simulink model "Furuta_Template_s"  (Simulink 10.0)
settings: Solver=ode4  StartTime=0.0  StopTime=50  FixedStep=0.0001  RelTol=1e-8  EnableMultiTasking=on
values from neighbouring files (symbols this model uses):
  b1 = 10^-4    (= 0.0001)    [SystemParameters.m]    (also in changeable_parameters.m)
  b2 = 2.8*(10^-4)    (= 0.00028)    [SystemParameters.m]    (also in changeable_parameters.m)
  g = 9.8    [SystemParameters.m]
  J2Hat = J2 + M2*((l2)^2)    (= 0.0055028)    [SystemParameters.m]
  JNotHat = J1Hat + M2*((L1)^2)    (= 0.0373463)    [SystemParameters.m]
  Km = 0.09    [SystemParameters.m]    (also in changeable_parameters.m)
  L = 0.005    [SystemParameters.m]    (also in changeable_parameters.m)
  L1 = 0.278    [SystemParameters.m]    (also in changeable_parameters.m)
  l2 = 0.148    [SystemParameters.m]    (also in changeable_parameters.m)
  M2 = 0.075    [SystemParameters.m]
  R = 7.8    [SystemParameters.m]    (also in changeable_parameters.m = B_mod'*Rh*Rh*B_mod)
  theta2_Init = pi +0.1    (= 3.24159265359)    [SystemParameters.m]
settings Model: Creator=mecmg  LastModifiedBy=Owner
settings DataIOCC: LimitDataPoints=on  SignalLoggingSaveFormat=ModelDataLogs
settings OptimizationCC: ExpressionDepthLimit=2147483647
settings DebuggingCC: SolverPrmCheckMsg=warning  FcnCallInpInsideContextMsg=warning  StateNameClashWarn=warning
settings GRTTargetCC: GeneratePreprocessorConditionals=Disable all
settings ConfigComp: CovExternalEMLEnable=off

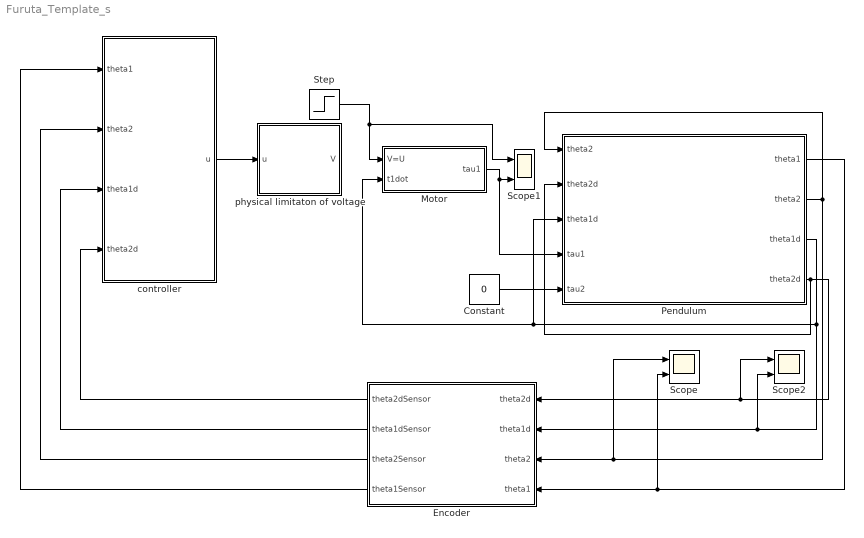
== system Furuta_Template_s ==
  Constant : Constant  Value=0  VectorParams1D=off
  Encoder : Subsystem
  Motor : Subsystem
  Pendulum : Subsystem
  Scope : Scope  NumInputPorts=2
  Scope1 : Scope  NumInputPorts=2
  Scope2 : Scope  NumInputPorts=2
  Step : Step  After=-10  SampleTime=0
  controller : Subsystem
  physical limitaton of voltage : Subsystem
  wires:
  controller/1(u) -> physical limitaton of voltage/1(u)
  Encoder/1(theta2dSensor) -> controller/4(theta2d)
  Encoder/4(theta1Sensor) -> controller/1(theta1)
  Encoder/2(theta1dSensor) -> controller/3(theta1d)
  Encoder/3(theta2Sensor) -> controller/2(theta2)
  Pendulum/2(theta2) -> Encoder/3(theta2), Scope/1, Pendulum/1("theta2  ")
  Pendulum/1(theta1) -> Encoder/4(theta1), Scope/2
  Pendulum/3(theta1d) -> Motor/2(t1dot), Pendulum/3("theta1d "), Scope2/2, Encoder/2(theta1d)
  Pendulum/4(theta2d) -> Pendulum/2("theta2d "), Scope2/1, Encoder/1(theta2d)
  Constant/1 -> Pendulum/5(tau2)
  Step/1 -> Scope1/1, Motor/1(V=U)
  Motor/1(tau1) -> Scope1/2, Pendulum/4(tau1)

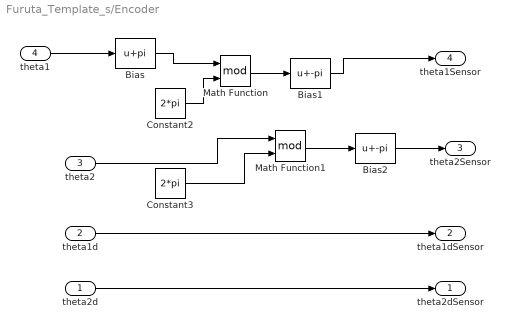
== system Furuta_Template_s/Encoder ==
  theta2d : Inport
  theta1d : Inport  Port=2
  theta2 : Inport  Port=3
  theta1 : Inport  Port=4
  Bias : Bias  Bias=pi
  Bias1 : Bias  Bias=-pi
  Bias2 : Bias  Bias=-pi
  Constant2 : Constant  Value=2*pi
  Constant3 : Constant  Value=2*pi
  Math Function : Math  Operator=mod  SignedPower=off  SaturateOnIntegerOverflow=on
  Math Function1 : Math  Operator=mod  SignedPower=off  SaturateOnIntegerOverflow=on
  theta2dSensor : Outport
  theta1dSensor : Outport  Port=2
  theta2Sensor : Outport  Port=3
  theta1Sensor : Outport  Port=4
  wires:
  theta1d/1 -> theta1dSensor/1
  theta2d/1 -> theta2dSensor/1
  theta1/1 -> Bias/1
  Constant2/1 -> Math Function/2
  Math Function/1 -> Bias1/1
  Math Function1/1 -> Bias2/1
  Constant3/1 -> Math Function1/2
  theta2/1 -> Math Function1/1
  Bias/1 -> Math Function/1
  Bias1/1 -> theta1Sensor/1
  Bias2/1 -> theta2Sensor/1

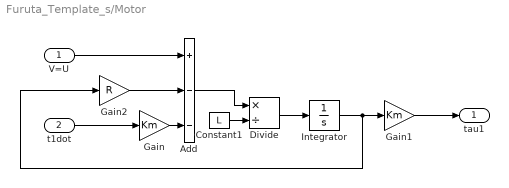
== system Furuta_Template_s/Motor ==
  V=U : Inport
  t1dot : Inport  Port=2
  Add : Sum  Inputs=+--
  Constant1 : Constant  Value=L
  Divide : Product  Inputs=*/
  Gain : Gain  Gain=Km
  Gain1 : Gain  Gain=Km
  Gain2 : Gain  Gain=R
  Integrator : Integrator
  tau1 : Outport
  wires:
  V=U/1 -> Add/1
  Gain2/1 -> Add/2
  t1dot/1 -> Gain/1
  Gain/1 -> Add/3
  Add/1 -> Divide/1
  Constant1/1 -> Divide/2
  Divide/1 -> Integrator/1
  Integrator/1 -> Gain2/1, Gain1/1
  Gain1/1 -> tau1/1

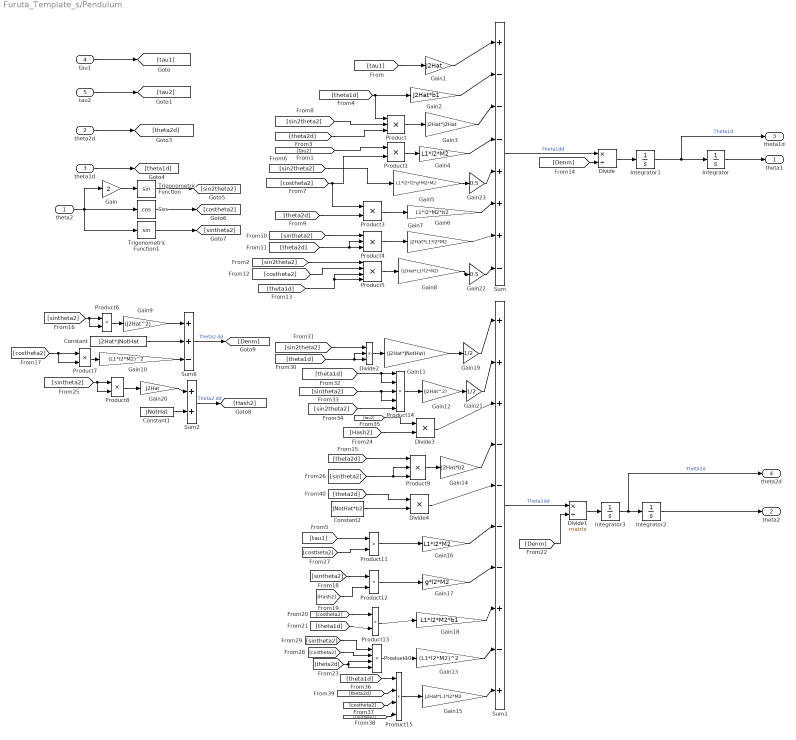
== system Furuta_Template_s/Pendulum ==
  "theta2  " : Inport
  "theta2d " : Inport  Port=2
  "theta1d " : Inport  Port=3
  tau1 : Inport  Port=4
  tau2 : Inport  Port=5
  Constant : Constant  Value=J2Hat*JNotHat
  Constant1 : Constant  Value=JNotHat
  Constant2 : Constant  Value=JNotHat*b2
  Cos : Trigonometry  Operator=cos
  Divide : Product  Inputs=*/
  Divide1 : Product  Inputs=*/  Multiplication=Matrix(*)
  Divide2 : Product  Inputs=***
  Divide3 : Product
  Divide4 : Product
  Gain : Gain  Gain=2
  Gain1 : Gain  Gain=J2Hat
  Gain10 : Gain  Gain=(L1*l2*M2)^2
  Gain11 : Gain  Gain=(J2Hat*JNotHat)
  Gain12 : Gain  Gain=(J2Hat^2)
  Gain13 : Gain  Gain=(L1*l2*M2)^2
  Gain14 : Gain  Gain=J2Hat*b2
  Gain15 : Gain  Gain=J2Hat*L1*l2*M2
  Gain16 : Gain  Gain=L1*l2*M2
  Gain17 : Gain  Gain=g*l2*M2
  Gain18 : Gain  Gain=L1*l2*M2*b1
  Gain19 : Gain  Gain=1/2
  Gain2 : Gain  Gain=J2Hat*b1
  Gain20 : Gain  Gain=J2Hat
  Gain21 : Gain  Gain=1/2
  Gain22 : Gain  Gain=0.5
  Gain23 : Gain  Gain=0.5
  Gain3 : Gain  Gain=J2Hat*J2Hat
  Gain4 : Gain  Gain=L1*l2*M2
  Gain5 : Gain  Gain=L1*l2*l2*g*M2*M2
  Gain6 : Gain  Gain=L1*l2*M2*b2
  Gain7 : Gain  Gain=J2Hat*L1*l2*M2
  Gain8 : Gain  Gain=(J2Hat*L1*l2*M2)
  Gain9 : Gain  Gain=(J2Hat^2)
  Integrator : Integrator  UpperSaturationLimit=pi  LowerSaturationLimit=-pi
  Integrator1 : Integrator
  Integrator2 : Integrator  InitialCondition=theta2_Init  UpperSaturationLimit=pi  LowerSaturationLimit=-pi
  Integrator3 : Integrator
  Product : Product  Inputs=3
  Product{1,3,6..8,11..13} (8 alike) : Product
  Product10 : Product  Inputs=4
  Product14 : Product  Inputs=5
  Product15 : Product  Inputs=4
  Product4 : Product  Inputs=3
  Product5 : Product  Inputs=4
  Product9 : Product  Inputs=3
  Sum : Sum  Inputs=|+---+++-
  Sum1 : Sum  Inputs=|+++----+-+
  Sum2 : Sum
  Sum6 : Sum  Inputs=++-
  Trigonometric Function : Trigonometry
  Trigonometric Function1 : Trigonometry
  theta1 : Outport
  theta2 : Outport  Port=2
  theta1d : Outport  Port=3
  theta2d : Outport  Port=4
  wires:
  Integrator1/1 -> Integrator/1, theta1d/1  "Theta1d"
  Integrator/1 -> theta1/1
  tau2/1 -> [tau2]
  tau1/1 -> [tau1]
  Integrator2/1 -> theta2/1
  "theta2  "/1 -> Gain/1, Trigonometric Function1/1, Cos/1
  Gain/1 -> Trigonometric Function/1
  Trigonometric Function/1 -> [sin2theta2]
  Cos/1 -> [costheta2]
  Trigonometric Function1/1 -> [sintheta2]
  "theta1d "/1 -> [theta1d]
  "theta2d "/1 -> [theta2d]
  Gain1/1 -> Sum/1
  [tau1] -> Gain1/1
  [theta1d] -> Product/1, Gain2/1
  Gain2/1 -> Sum/2
  Product/1 -> Gain3/1
  [sin2theta2] -> Product/2
  [theta2d] -> Product/3
  Gain3/1 -> Sum/3
  Gain4/1 -> Sum/4
  Product1/1 -> Gain4/1
  [costheta2] -> Product3/1, Product1/2
  [tau2] -> Product1/1
  [sin2theta2] -> Gain5/1
  Product3/1 -> Gain6/1
  [theta2d] -> Product3/2
  [sintheta2] -> Product4/1
  [theta2d] -> Product4/3, Product4/2
  Product4/1 -> Gain7/1
  Product5/1 -> Gain8/1
  [sin2theta2] -> Product5/1
  [costheta2] -> Product5/2
  [theta1d] -> Product5/4, Product5/3
  Sum6/1 -> [Denm]  "Theta2 dd"
  Gain9/1 -> Sum6/1
  Constant/1 -> Sum6/2
  Gain10/1 -> Sum6/3
  Product6/1 -> Gain9/1
  Product7/1 -> Gain10/1
  [costheta2] -> Product7/2, Product7/1
  [sintheta2] -> Product6/2, Product6/1
  Sum/1 -> Divide/1  "Theta1dd"
  [Denm] -> Divide/2
  Divide/1 -> Integrator1/1
  Divide1/1 -> Integrator3/1
  [Denm] -> Divide1/2
  Sum1/1 -> Divide1/1  "Theta2dd"
  Product13/1 -> Gain18/1
  Gain18/1 -> Sum1/8
  Product12/1 -> Gain17/1
  [Hash2] -> Product12/2
  [sintheta2] -> Product12/1
  Gain17/1 -> Sum1/7
  Product11/1 -> Gain16/1
  Product9/1 -> Gain14/1
  Gain14/1 -> Sum1/4
  Gain12/1 -> Gain21/1
  Integrator3/1 -> theta2d/1, Integrator2/1  "Theta2d"
  Divide2/1 -> Gain11/1
  [theta1d] -> Divide2/2, Divide2/3
  [sin2theta2] -> Divide2/1
  [theta1d] -> Product14/2, Product14/1
  [sintheta2] -> Product14/4, Product14/3
  [sin2theta2] -> Product14/5
  Product14/1 -> Gain12/1
  [sintheta2] -> Product8/1, Product8/2
  Product8/1 -> Gain20/1
  Constant1/1 -> Sum2/2
  Gain20/1 -> Sum2/1
  Sum2/1 -> [Hash2]  "Theta2 dd"
  [tau2] -> Divide3/1
  [Hash2] -> Divide3/2
  Divide3/1 -> Sum1/3
  [sintheta2] -> Product9/2, Product9/3
  [theta2d] -> Product9/1
  Gain16/1 -> Sum1/6
  [tau1] -> Product11/1
  [costheta2] -> Product11/2
  [costheta2] -> Product13/1
  [theta1d] -> Product13/2
  Gain13/1 -> Sum1/9
  Product10/1 -> Gain13/1
  [costheta2] -> Product10/2
  [sintheta2] -> Product10/1
  Gain15/1 -> Sum1/10
  Product15/1 -> Gain15/1
  [theta1d] -> Product15/1
  [theta2d] -> Product10/4, Product10/3
  [costheta2] -> Product15/3
  [sin2theta2] -> Product15/4
  [theta2d] -> Product15/2
  Gain11/1 -> Gain19/1
  Gain19/1 -> Sum1/1
  Gain21/1 -> Sum1/2
  Gain8/1 -> Gain22/1
  Gain22/1 -> Sum/8
  Divide4/1 -> Sum1/5
  Constant2/1 -> Divide4/2
  [theta2d] -> Divide4/1
  Gain5/1 -> Gain23/1
  Gain6/1 -> Sum/6
  Gain7/1 -> Sum/7
  Gain23/1 -> Sum/5

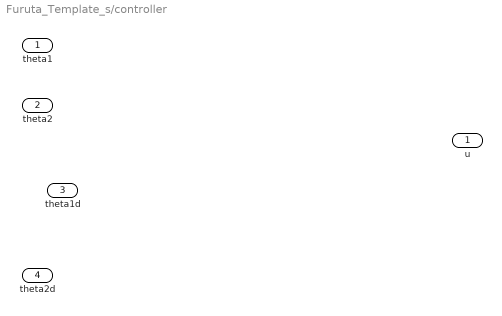
== system Furuta_Template_s/controller ==
  theta1 : Inport
  theta2 : Inport  Port=2
  theta1d : Inport  Port=3
  theta2d : Inport  Port=4
  u : Outport

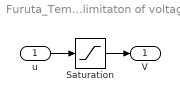
== system Furuta_Template_s/physical limitaton of voltage ==
  u : Inport
  Saturation : Saturate  UpperLimit=10  LowerLimit=0
  V : Outport
  wires:
  u/1 -> Saturation/1
  Saturation/1 -> V/1
